simulink model "nonlinear_resistor"  (R2014a)
settings: Solver=VariableStepDiscrete  StartTime=0.0  StopTime=20/60  RelTol=1e-3
PreLoadFcn:
  | load('nlResistor_data');
values from neighbouring files (symbols this model uses):
  nlResistor_I = [-30 -30 -30 -30 -30 -30 -30 -30 -30 -30 -30 -30 ... (141 elements, 1x141)]    [nlResistor_data.mat]
  nlResistor_V = [-70 -69 -68 -67 -66 -65 -64 -63 -62 -61 -60 -59 ... (141 elements, 1x141)]    [nlResistor_data.mat]
libraries: powerlib x6, simulink x1
settings Model: Creator=gdudgeon  LastModifiedBy=cosorio
settings DataIOCC: SignalLoggingSaveFormat=ModelDataLogs  SaveOutput=off  SaveTime=off
settings OptimizationCC: ExpressionDepthLimit=2147483647
settings DebuggingCC: UnderspecifiedInitializationDetection=Classic  FcnCallInpInsideContextMsg=UseLocalSettings  StateNameClashWarn=warning
settings GRTTargetCC: CombineOutputUpdateFcns=off  GRTInterface=on

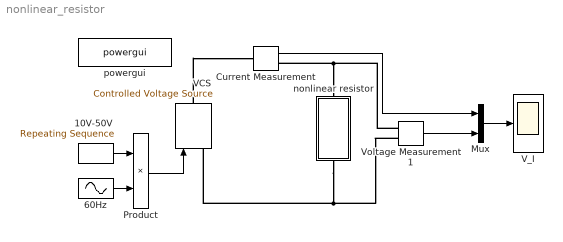
== system nonlinear_resistor ==
  10V-50V : simulink/Sources/Repeating Sequence  rep_seq_t=[0 5/60 15/60 20/60]  rep_seq_y=[10 10 50 50]
  60Hz : Sin  Frequency=2*pi*60  SampleTime=0
  Current Measurement : powerlib/Measurements/Current Measurement  PhasorSimulation=off  OutputType=Complex  PSBequivalent=0
  Mux : Mux  Inputs=2
  Product : Product  RndMeth=Zero
  VCS : powerlib/Electrical Sources/Controlled Voltage Source  Initialize=on  Source_Type=AC  Amplitude=0  Phase=0  Frequency=0  Measurements=None
  V_I : Scope
      settings: YMin=-60  YMax=60  SaveName=VI
  Voltage Measurement1 : powerlib/Measurements/Voltage Measurement  PhasorSimulation=off  OutputType=Complex  PSBequivalent=0
  nonlinear resistor : Subsystem
  powergui : powerlib/powergui  SimulationMode=Discrete  SolverType=Tustin  SampleTime=2e-5  frequency=60  SPID=off  DisableSnubberDevices=off  DisableRonSwitches=off  DisableVfSwitches=off  SwTol=0  Interpol=off  DisplayEquations=off  Ts=0  methode=off  frequencyindice=0  Pbase=100e6  ErrMax=1e-4  Iterations=50  UnitsV=kV  UnitsW=MW  FunctionMessages=off  echomessages=off  HookPort=off  EnableUseOfTLC=off  x0status=blocks  RestoreLinks=warning  ResistiveCurrentMeasurement=off  Frange=[0:2:500]  Ylog=off  Xlog=on  ShowGrid=off  save=off  variable=ZData  structure=0  ZoomFFT=on  StartTime=0.0  cycles=1  DisplayStyle=1  fundamental=60  FreqAxis=off  MaxFrequency=1000  frequencyindicesteady=1  RmsSteady=1  display=off
  wires:
  Product/1 -> VCS/1
  60Hz/1 -> Product/2
  10V-50V/1 -> Product/1
  Mux/1 -> V_I/1
  Voltage Measurement1/1 -> Mux/2
  Current Measurement/1 -> Mux/1
  connections:
  VCS/RConn1 -- Current Measurement/LConn1
  Voltage Measurement1/LConn1 -- Current Measurement/RConn1 -- nonlinear resistor/LConn1
  Voltage Measurement1/LConn2 -- VCS/LConn1 -- nonlinear resistor/RConn1

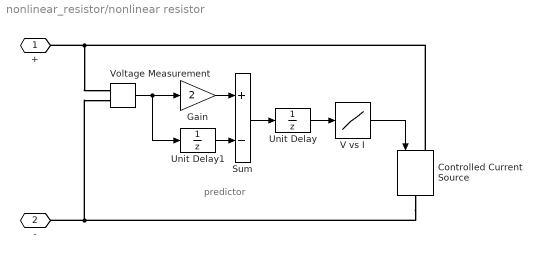
== system nonlinear_resistor/nonlinear resistor ==
  note: predictor
  Controlled Current Source : powerlib/Electrical Sources/Controlled Current Source  Initialize=on  Source_Type=AC  Amplitude=0  Phase=0  Frequency=0  Measurements=None
  Gain : Gain  Gain=2
  Sum : Sum  Inputs=+-
  Unit Delay : UnitDelay  SampleTime=-1
  Unit Delay1 : UnitDelay  SampleTime=-1
  V vs I : Lookup  InputValues=nlResistor_V  Table=nlResistor_I
  Voltage Measurement : powerlib/Measurements/Voltage Measurement  PhasorSimulation=off  OutputType=Complex  PSBequivalent=0
  + : PMIOPort  Port=1  Side=Left
  - : PMIOPort  Port=2  Side=Right
  wires:
  V vs I/1 -> Controlled Current Source/1
  Unit Delay/1 -> V vs I/1
  Sum/1 -> Unit Delay/1
  Voltage Measurement/1 -> Gain/1, Unit Delay1/1
  Unit Delay1/1 -> Sum/2
  Gain/1 -> Sum/1
  connections:
  Controlled Current Source/LConn1 -- +/RConn1 -- Voltage Measurement/LConn1
  Controlled Current Source/RConn1 -- -/RConn1 -- Voltage Measurement/LConn2
